simulink model "QuadDynamics"  (R2016b)
settings: Solver=VariableStepAuto  StartTime=0.0  StopTime=100.0  RelTol=1e-3
settings Model: Creator=root  LastModifiedBy=root

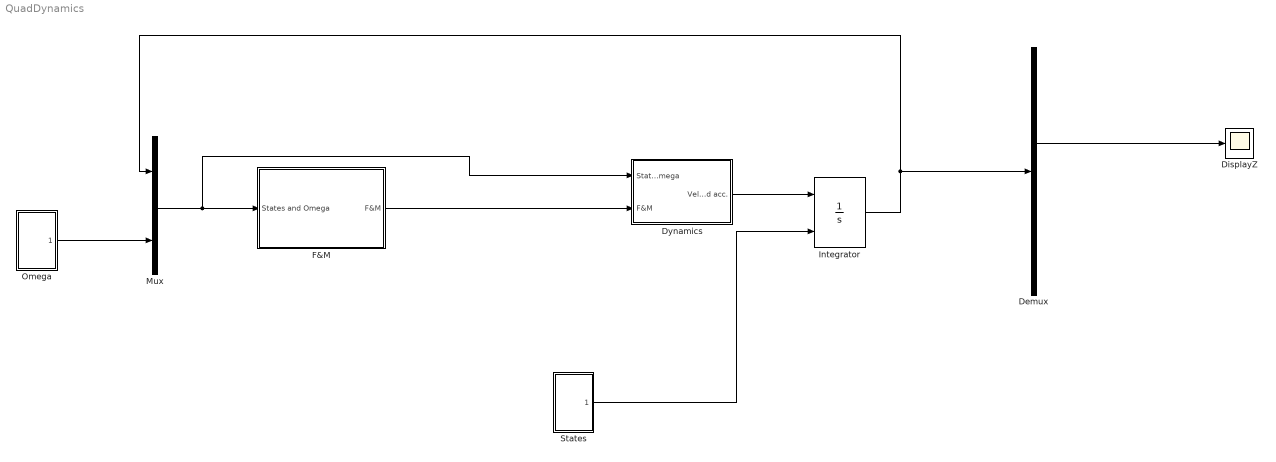
== system QuadDynamics ==
  Demux : Demux  Outputs=12
  DisplayZ : Scope
  Dynamics : Subsystem
  F&M : Subsystem
  Integrator : Integrator  InitialConditionSource=external
  Mux : Mux  Inputs=2
  Omega : Subsystem
  States : Subsystem
  wires:
  F&M/1(F&M) -> Dynamics/2(F&M)
  Integrator/1 -> Mux/1, Demux/1
  Demux/5 -> DisplayZ/1
  States/1("States ") -> Integrator/2
  Omega/1("Omega ") -> Mux/2
  Mux/1 -> Dynamics/1(States and Omega), F&M/1(States and Omega)
  Dynamics/1("Velocity and acc. ") -> Integrator/1

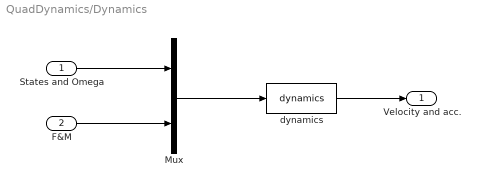
== system QuadDynamics/Dynamics ==
  States and Omega : Inport
  F&M : Inport  Port=2
  Mux : Mux  Inputs=2
  dynamics : MATLABFcn  MATLABFcn=dynamics  OutputDimensions=12
  "Velocity and acc. " : Outport
  wires:
  Mux/1 -> dynamics/1
  F&M/1 -> Mux/2
  States and Omega/1 -> Mux/1
  dynamics/1 -> "Velocity and acc. "/1

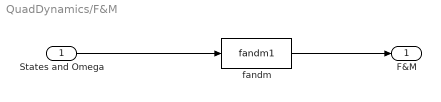
== system QuadDynamics/F&M ==
  States and Omega : Inport
  fandm : MATLABFcn  MATLABFcn=fandm1  OutputDimensions=24
  F&M : Outport
  wires:
  fandm/1 -> F&M/1
  States and Omega/1 -> fandm/1

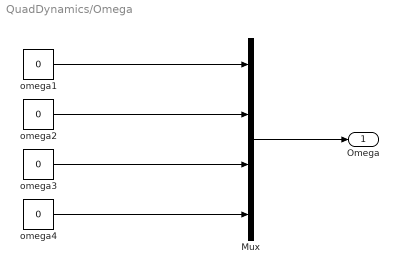
== system QuadDynamics/Omega ==
  Mux : Mux
  omega{1..4} (4 alike) : Constant  Value=0
  "Omega " : Outport
  wires:
  Mux/1 -> "Omega "/1
  omega3/1 -> Mux/3
  omega4/1 -> Mux/4
  omega1/1 -> Mux/1
  omega2/1 -> Mux/2

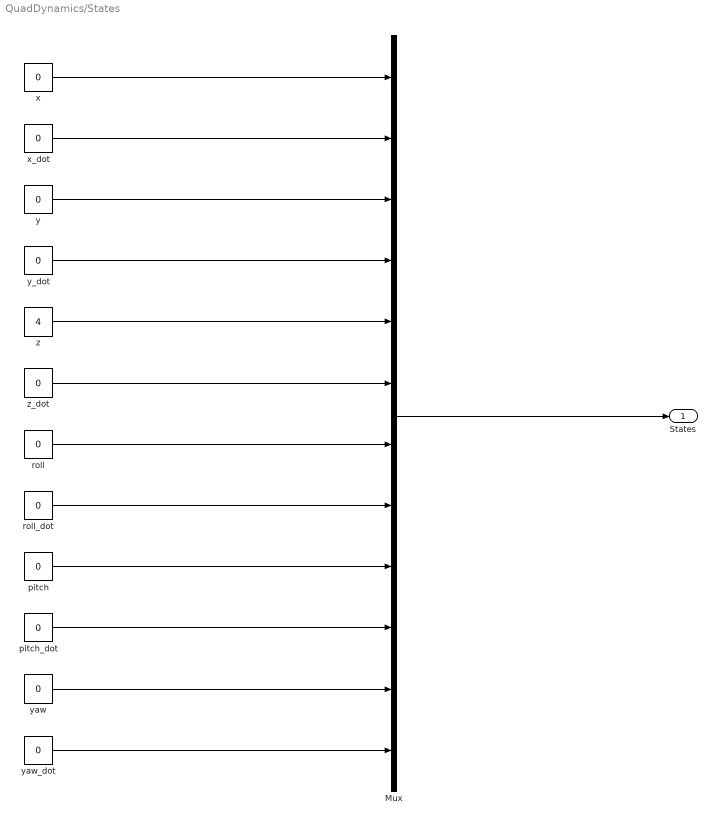
== system QuadDynamics/States ==
  Mux : Mux  Inputs=12
  pitch : Constant  Value=0
  pitch_dot : Constant  Value=0
  roll : Constant  Value=0
  roll_dot : Constant  Value=0
  x : Constant  Value=0
  x_dot : Constant  Value=0
  y : Constant  Value=0
  y_dot : Constant  Value=0
  yaw : Constant  Value=0
  yaw_dot : Constant  Value=0
  z : Constant  Value=4
  z_dot : Constant  Value=0
  "States " : Outport
  wires:
  y/1 -> Mux/3
  z/1 -> Mux/5
  z_dot/1 -> Mux/6
  x/1 -> Mux/1
  pitch_dot/1 -> Mux/10
  x_dot/1 -> Mux/2
  roll/1 -> Mux/7
  yaw/1 -> Mux/11
  y_dot/1 -> Mux/4
  pitch/1 -> Mux/9
  roll_dot/1 -> Mux/8
  yaw_dot/1 -> Mux/12
  Mux/1 -> "States "/1
